simulink model "PMSM3P2LInverterCHILsystem"  (R2026a)
settings: Solver=FixedStepAuto  StopTime=inf  FixedStep=Ts_CPU  EnableMultiTasking=on
undefined symbols (not defined in the file): DiscIntNeverNeededParam, F28379D_ADC_MaxCount, F28379D_ADC_Vmax, Foc_Ki_IxTcpu, Foc_Ki_S, Foc_Kp_I, Foc_Kp_S, Ia_offset, Ib_offset, IO334, IO334_DAC_Vmax, IO334_iDAC_bias, IO334_iDAC_gain, Maxon_645604_J, Maxon_645604_lambda_pm, Maxon_645604_Ld, Maxon_645604_Lq, Maxon_645604_Np, Maxon_645604_Rs, Maxon_645604_StaticF, Maxon_645604_ViscousF, Maxon_Mile_Nslits, PMSM3P2LInverter_limited, PMSM_3P2L_Inverter_Plant, PU_System_I_base, PU_System_N_base, PWM_frequency, Ts_CAN_Tx, Ts_CPU, ts_FPGA_mdl, Ts_UI
libraries: speedgoatlib_hdlCoder_IO3xx x31, mcbcontrolslib x8, canmsglib x6, speedgoatlib_IO611 x3, mcbeeMathTransformLib x3, slpidlib x3, simulink x3, mcbpositiondecoderlib x3, pwm_cpulib x2, mcbhdlplantlib x2, demo_controls x1, quadrature_cpulib x1
(part 1 of 3)
settings Model: DataDictionary=PMSM3P2LInverterDd.sldd  EnableAccessToBaseWorkspace=off  SimulationMode=external  ExtModeEnableFloating=off  Creator=chrisz  LastModifiedBy=mathieu.lu-dac
settings SolverCC: ConcurrentTasks=on  PositivePriorityOrder=on
settings OptimizationCC: ConditionallyExecuteInputs=off  OptimizeBlockIOStorage=off
settings DebuggingCC: AlgebraicLoopMsg=error  SingleTaskRateTransMsg=error  TasksWithSamePriorityMsg=none  ParameterOverflowMsg=warning  ParameterUnderflowMsg=error  FixptConstUnderflowMsg=error  FixptConstOverflowMsg=error
settings HardwareCC: ProdBitPerLong=64.0  ProdHWDeviceType=Intel->x86-64 (Linux 64)  TargetBitPerPointer=64.0  TargetBitPerSizeT=64.0  TargetBitPerPtrDiffT=64.0  TargetLongLongMode=on  TargetIntDivRoundTo=Zero  TargetEndianess=LittleEndian  TargetWordSize=64.0  TargetHWDeviceType=Custom Processor->MATLAB Host Computer
settings RTWCC: SystemTargetFile=speedgoat.tlc  TemplateMakefile=slrealtime_default_tmf  Toolchain=Simulink Real-Time Toolchain  BuildConfiguration=Faster Runs  TargetLang=C++  Description=Speedgoat Real-Time Target Machine
settings SimulinkRealTimeTargetCC: SLRTFileLogMaxRuns=1.0  MultiwordLength=2048.0
settings SimscapeCC: SimscapeNominalValues="[{\"value\":\"1\",\"unit\":\"A\"},{\"value\":\"1\",\"unit\":\"bar\"},{\"value\":\"1\",\"unit\":\"cm^2\"},{\"value\":\"1\",\"unit\":\"cm^3/s\"},{\"value\":\"1\",\"unit\":\"kJ/kg\"},{\"value\":\"1\",\"unit\":\"kW\"},{\"value\":\"1\",\"unit\":\"l\"},{\"value\":\"1\",\"unit\":\"N\"},{\"value\":\"1\",\"unit\":\"N*m\"},{\"value\":\"1\",\"unit\":\"V\"}]"  SimscapeLogType=none  SimscapeLogDataHistory=5000.0

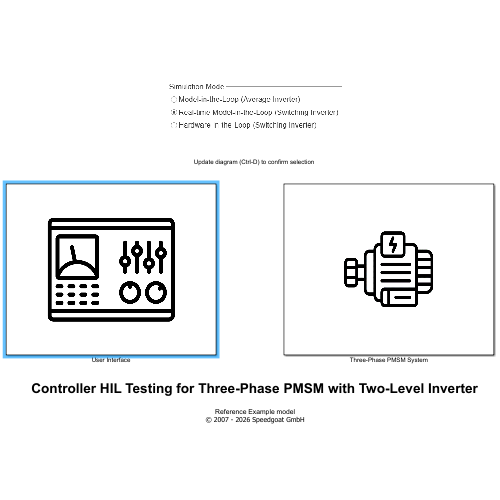
[thumbnail: Simulink's stored preview of the top-level diagram]
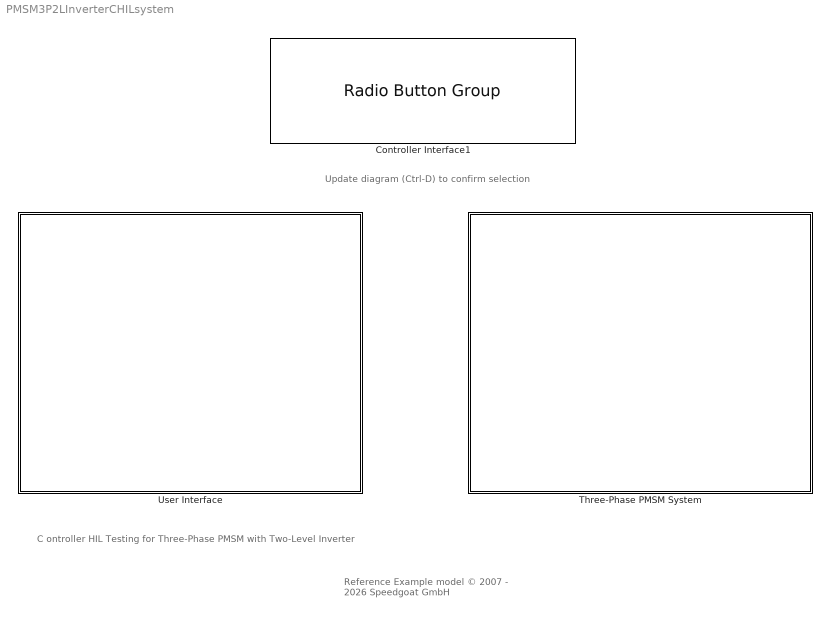
== system PMSM3P2LInverterCHILsystem ==
  note: Update diagram (Ctrl-D) to confirm selection
  note: Reference Example model
      | © 2007 - 2026 Speedgoat GmbH
  note: C ontroller HIL Testing for Three-Phase PMSM with Two-Level Inverter
  Controller Interface1 : RadioButtonGroup  LabelPosition=Hide  SelectedLabel=Real-time Model-in-the-Loop (Switching Inverter)  ButtonGroupName=Simulation Mode
  Three-Phase PMSM System : Subsystem
      mask Display: image('pmsmMask.png'); % Use "Edit Image" on toolstrip to change.
  User Interface : Subsystem
      mask Display: image('UIMask.png');

== system PMSM3P2LInverterCHILsystem/Three-Phase PMSM System ==
  Closed_Loop_FOC : Constant  OutDataTypeStr=boolean  SampleTime=Ts_UI
  Controller : Subsystem  Variant=on  VariantControl=Choice
      settings: PortSchema="{\"entries\":[{\"content\":{\"sides\":[{\"content\":{\"connectorIds\":[\"In1\",\"In2\",\"In3\",\"In4\",\"In5\",\"In6\"]},\"type\":\"ConnectorPlacement.EquallySpacedRectSide\",\"uuid\":\"39f08c92-b87f-4f95-877f-fef0e466fbdb\"},{\"content\":{\"connectorIds\":[\"Out1\"],\"side\":\"RIGHT\"},\"type\":\"ConnectorPlacement.EquallySpacedRectSide\",\"uuid\":\"6fadd6f2-7db3-41c1-89a7-be1692c18c49\"},{\"content\":{\"connectorIds\":[\"Out2\"],\"side\":\"TOP\"},\"type\":\"ConnectorPlacement.EquallySpacedRectSide\",\"uuid\":\"aea4ee68-7094-4bdc-b416-2d8969306971\"}]},\"type\":\"ConnectorPlacement.EquallySpacedConnector\",\"uuid\":\"e129f01f-1291-4735-8ea4-164650c1b4f8\"}],\"packageUris\":[\"http://schema.mathworks.com/mf0/Connector/R2020b\"],\"version\":\"1.0\"}"
      mask Display: image('MCUMask.png');
  Controller Parameters : Subsystem
  Controller_fbk_signals : Subsystem
  EnablePWM : Constant  OutDataTypeStr=boolean  SampleTime=Ts_UI
  Fault Trigering : Subsystem
  Load : Constant  Value=0  OutDataTypeStr=single
  Motor Model Feedback : Subsystem
  Mux : Mux  Inputs=2
  SimulationVariant : Constant  Value=2
  Speed_Cmd_rpm : Constant  Value=500  OutDataTypeStr=single  SampleTime=Ts_UI
  Terminator : Terminator
  Terminator2 : Terminator
  Three-Phase PMSM Drive : Subsystem  Variant=on  VariantControl=Choice
      settings: PortSchema="{\"entries\":[{\"content\":{\"sides\":[{\"content\":{\"connectorIds\":[\"In1\",\"In2\",\"In3\"]},\"type\":\"ConnectorPlacement.EquallySpacedRectSide\",\"uuid\":\"be3bef0c-fa0d-49a9-8d81-4a9438f9f09e\"},{\"content\":{\"connectorIds\":[\"Out1\",\"Out2\",\"Out3\",\"Out4\",\"Out5\",\"Out6\"],\"side\":\"RIGHT\"},\"type\":\"ConnectorPlacement.EquallySpacedRectSide\",\"uuid\":\"a97c4291-bd47-47ae-a87a-e148291abc4a\"},{\"content\":{\"connectorIds\":[\"In4\"],\"side\":\"TOP\"},\"type\":\"ConnectorPlacement.EquallySpacedRectSide\",\"uuid\":\"93bcf0c4-5b44-4ac3-b6c3-6b4577237bd1\"}]},\"type\":\"ConnectorPlacement.EquallySpacedConnector\",\"uuid\":\"9c4ab161-5f4a-4191-8213-47b9045836c1\"}],\"packageUris\":[\"http://schema.mathworks.com/mf0/Connector/R2020b\"],\"version\":\"1.0\"}"
      mask Display: image('pmsmMask.png'); % Use "Edit Image" on toolstrip to change.
  Voltage : Constant  Value=24  OutDataTypeStr=single
  wires:
  Controller/2(Simu_config) -> Three-Phase PMSM Drive/4(Simu_config)
  Voltage/1 -> Three-Phase PMSM Drive/1(V_dc)
  [Iab] -> Controller/1(Iab)
  Closed_Loop_FOC/1 -> Controller/4(Closed_Loop_FOC)
  Controller Parameters/1(Controller Parameters) -> Controller/6(Controller_Parameters)
  Load/1 -> Three-Phase PMSM Drive/3(LdTrq/Spd)
  [QAE_Pos_C] -> Controller/2(QAE_MIL_fbk)
  Mux/1 -> [Iab]
  Fault Trigering/1(Faults) -> Three-Phase PMSM Drive/2(Fault)
  Controller/1(Controller_fbk) -> Controller_fbk_signals/1(Controller_fbk)
  Three-Phase PMSM Drive/1(Ia) -> Mux/1, Motor Model Feedback/1(Ia)
  Three-Phase PMSM Drive/2(Ib) -> Mux/2, Motor Model Feedback/2(Ib)
  Three-Phase PMSM Drive/3(Ic) -> Motor Model Feedback/3(Ic)
  Three-Phase PMSM Drive/4(Motor_Spd) -> Motor Model Feedback/4(Motor_SPD_rads)
  Three-Phase PMSM Drive/6(QAE_Pos_C) -> [QAE_Pos_C]
  Three-Phase PMSM Drive/5(Motor_Angle) -> Terminator/1
  EnablePWM/1 -> Controller/3(EnablePWM)
  Speed_Cmd_rpm/1 -> Controller/5(Speed_CMD_RPM)
  SimulationVariant/1 -> Terminator2/1

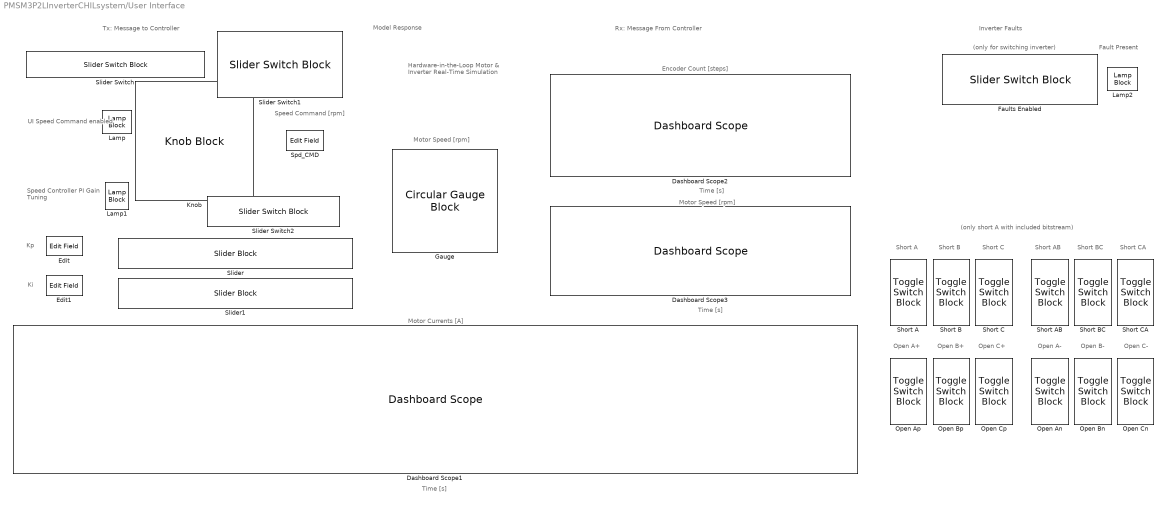
== system PMSM3P2LInverterCHILsystem/User Interface ==
  note: Fault Present
  note: Hardware-in-the-Loop
      | Motor & Inverter
      | Real-Time Simulation
  note: Motor Currents [A]
  note: Model Response
  note: Kp
  note: UI Speed Command
      | enabled
  note: Tx: Message to Controller
  note: Speed Controller
      | PI Gain Tuning
  note: Ki
  note: Rx: Message From Controller
  note: Open A-
  note: Open C-
  note: Short AB
  note: Short B
  note: Short CA
  note: Open A+
  note: Short BC
  note: Open B-
  note: Open B+
  note: Open C+
  note: Short A
  note: Short C
  note: Inverter Faults
  note: Motor Speed [rpm]
  note: Time [s]
  note: Time [s]
  note: Time [s]
  note: Motor Speed [rpm]
  note: Encoder Count [steps]
  note: Speed Command [rpm]
  note: (only for switching inverter)
  note: (only short A with included bitstream)
  Dashboard Scope1 : DashboardScope  ShowInitialText=off  TimeSpan=0.10000000000000001  Ymin=-50  Ymax=50  ScaleAtStop=off  UpdateMode=Scroll  FontColor=[0.0, 0.0, 0.0]
  Dashboard Scope2 : DashboardScope  ShowInitialText=off  TimeSpan=1  Ymin=0  Ymax=1e5  ScaleAtStop=off  FontColor=[0.0, 0.0, 0.0]
  Dashboard Scope3 : DashboardScope  ShowInitialText=off  TimeSpan=10  Ymin=-1500  Ymax=1500  ScaleAtStop=off  FontColor=[0.0, 0.0, 0.0]
  Edit : EditField  LabelPosition=Hide  ShowInitialText=on  Alignment=Center
  Edit1 : EditField  LabelPosition=Hide  ShowInitialText=on  Alignment=Center
  Faults Enabled : SliderSwitchBlock  LabelPosition=Hide
  Gauge : CircularGaugeBlock  LabelPosition=Hide  ScaleMin=-1500  ScaleMax=1500  FontColor=[0.0, 0.0, 0.0]
  Knob : KnobBlock  LabelPosition=Hide  ScaleMin=-1500  ScaleMax=1500
  Lamp : LampBlock  LabelPosition=Hide  DefaultColor=[192.0, 192.0, 192.0]
  Lamp1 : LampBlock  LabelPosition=Hide  DefaultColor=[192.0, 192.0, 192.0]
  Lamp2 : LampBlock  LabelPosition=Hide  DefaultColor=[192.0, 192.0, 192.0]
  Open An : ToggleSwitchBlock  LabelPosition=Hide
  Open Ap : ToggleSwitchBlock  LabelPosition=Hide
  Open Bn : ToggleSwitchBlock  LabelPosition=Hide
  Open Bp : ToggleSwitchBlock  LabelPosition=Hide
  Open Cn : ToggleSwitchBlock  LabelPosition=Hide
  Open Cp : ToggleSwitchBlock  LabelPosition=Hide
  Short A : ToggleSwitchBlock  LabelPosition=Hide
  Short AB : ToggleSwitchBlock  LabelPosition=Hide
  Short B : ToggleSwitchBlock  LabelPosition=Hide
  Short BC : ToggleSwitchBlock  LabelPosition=Hide
  Short C : ToggleSwitchBlock  LabelPosition=Hide
  Short CA : ToggleSwitchBlock  LabelPosition=Hide
  Slider : SliderBlock  LabelPosition=Hide  ScaleMin=1e-5  ScaleMax=10  ScaleType=Log
  Slider Switch : SliderSwitchBlock  LabelPosition=Hide
  Slider Switch1 : SliderSwitchBlock  LabelPosition=Hide
  Slider Switch2 : SliderSwitchBlock  LabelPosition=Hide
  Slider1 : SliderBlock  LabelPosition=Hide  ScaleMin=1e-5  ScaleMax=10  ScaleType=Log
  Spd_CMD : EditField  LabelPosition=Hide  ShowInitialText=on  Alignment=Center

== system PMSM3P2LInverterCHILsystem/Three-Phase PMSM System/Controller ==
  Iab : Inport
  QAE_MIL_fbk : Inport  Port=2
  EnablePWM : Inport  Port=3
  Closed_Loop_FOC : Inport  Port=4
  Speed_CMD_RPM : Inport  Port=5
  Controller_Parameters : Inport  Port=6
  Controller_HIL_CAN : Subsystem  VariantControl=strcmp(get_param([bdroot '/Three-Phase PMSM System/SimulationVariant'], 'Value'),'3')
  Controller_MIL : Subsystem  VariantControl=(default)
  Controller_fbk : Outport
  Simu_config : Outport  Port=2

== system PMSM3P2LInverterCHILsystem/Three-Phase PMSM System/Controller Parameters ==
  Controller_Parameters : BusCreator  Inputs=6
  Controller_Parameters1 : BusCreator  Inputs=6
  Default Values : Constant  OutDataTypeStr=boolean  SampleTime=Ts_UI
  Foc_Ki_S : Constant  Value=Foc_Ki_S  OutDataTypeStr=single
  Foc_Kp_I : Constant  Value=Foc_Kp_I  OutDataTypeStr=single
  Foc_Kp_S : Constant  Value=Foc_Kp_S  OutDataTypeStr=single
  Ia Offset : Constant  Value=Ia_offset  OutDataTypeStr=single
  Ia_offset : Constant  Value=Ia_offset  OutDataTypeStr=single  SampleTime=Ts_UI
  Ib Offset : Constant  Value=Ib_offset  OutDataTypeStr=single
  Ib_offset : Constant  Value=Ib_offset  OutDataTypeStr=single  SampleTime=Ts_UI
  Ki_S : Constant  Value=0.1  OutDataTypeStr=single  SampleTime=Ts_UI
  Ki_i*Tcpu : Constant  Value=Foc_Ki_IxTcpu  OutDataTypeStr=single  SampleTime=Ts_UI
  Ki_i*Tcpu1 : Constant  Value=Foc_Ki_IxTcpu  OutDataTypeStr=single
  Kp_I : Constant  Value=Foc_Kp_I  OutDataTypeStr=single  SampleTime=Ts_UI
  Kp_S : Constant  Value=0.1  OutDataTypeStr=single  SampleTime=Ts_UI
  Rate Transition : RateTransition  OutPortSampleTime=Ts_UI
  Switch : Switch  Criteria=u2 ~= 0  SaturateOnIntegerOverflow=off  InputSameDT=off
  Controller Parameters : Outport
  wires:
  Ia_offset/1 -> Controller_Parameters/5  "Ia_offset"
  Foc_Kp_S/1 -> Controller_Parameters1/1  "Kp_S"
  Ia Offset/1 -> Controller_Parameters1/5  "Ia_offset"
  Ib Offset/1 -> Controller_Parameters1/6  "Ib_offset"
  Controller_Parameters/1 -> Switch/3
  Foc_Ki_S/1 -> Controller_Parameters1/2  "Ki_S"
  Foc_Kp_I/1 -> Controller_Parameters1/3  "Kp_I"
  Controller_Parameters1/1 -> Rate Transition/1
  Ib_offset/1 -> Controller_Parameters/6  "Ib_offset"
  Ki_i*Tcpu/1 -> Controller_Parameters/4  "Ki_IxTcpu"
  Ki_S/1 -> Controller_Parameters/2  "Ki_S"
  Ki_i*Tcpu1/1 -> Controller_Parameters1/4  "Ki_IxTcpu"
  Kp_I/1 -> Controller_Parameters/3  "Kp_I"
  Kp_S/1 -> Controller_Parameters/1  "Kp_S"
  Switch/1 -> Controller Parameters/1
  Rate Transition/1 -> Switch/1
  Default Values/1 -> Switch/2  "Default Values"

== system PMSM3P2LInverterCHILsystem/Three-Phase PMSM System/Controller_fbk_signals ==
  Controller_fbk : Inport
  Data Type Conversion : DataTypeConversion  OutDataTypeStr=boolean  SaturateOnIntegerOverflow=off  RndMeth=Floor
  Demux : Demux
  Terminator{,1..3} (4 alike) : Terminator
  wires:
  Demux/1 -> Terminator1/1  "Speed_fbk"
  Controller_fbk/1 -> Demux/1
  Demux/2 -> Terminator3/1  "Encoder_Pos_fbk"
  Demux/4 -> Data Type Conversion/1  "Spd_Pot_fdk"
  Demux/3 -> Terminator2/1  "Speed_Cmd_fbk"
  Data Type Conversion/1 -> Terminator/1  "Spd_pot_enable"

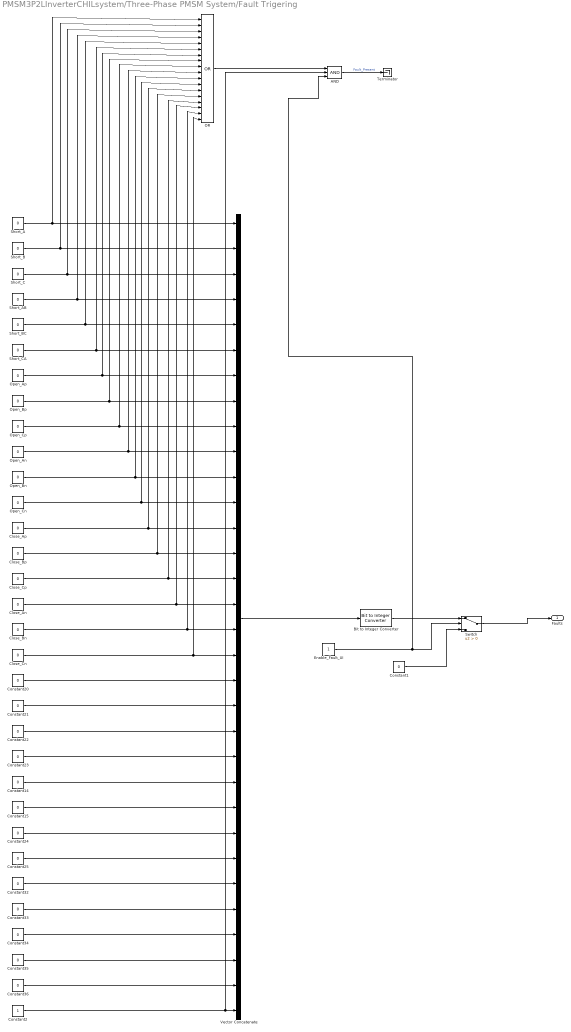
== system PMSM3P2LInverterCHILsystem/Three-Phase PMSM System/Fault Trigering ==
  AND : Logic  Inputs=3  IconShape=distinctive  AllPortsSameDT=off  OutDataTypeStr=boolean
  Bit to Integer Converter : simulink/Logic and Bit Operations/Bit to Integer Converter  nbits=32  bitOrder=LSB first  signedOutputValues=Unsigned  outDtype=uint32  outDtypeSigned=Inherit via internal rule
  Close_An : Constant  Value=0  OutDataTypeStr=boolean  SampleTime=Ts_UI
  Close_Ap : Constant  Value=0  OutDataTypeStr=boolean  SampleTime=Ts_UI
  Close_Bn : Constant  Value=0  OutDataTypeStr=boolean  SampleTime=Ts_UI
  Close_Bp : Constant  Value=0  OutDataTypeStr=boolean  SampleTime=Ts_UI
  Close_Cn : Constant  Value=0  OutDataTypeStr=boolean  SampleTime=Ts_UI
  Close_Cp : Constant  Value=0  OutDataTypeStr=boolean  SampleTime=Ts_UI
  Constant1 : Constant  Value=0  OutDataTypeStr=uint32
  Constant{14..15,20..25,32..36} (13 alike) : Constant  Value=0  OutDataTypeStr=boolean  SampleTime=Ts_UI
  Constant2 : Constant  OutDataTypeStr=boolean  SampleTime=Ts_UI
  Enable_Fault_UI : Constant  OutDataTypeStr=boolean  SampleTime=Ts_UI
  OR : Logic  Operator=OR  Inputs=18  IconShape=distinctive  AllPortsSameDT=off  OutDataTypeStr=boolean
  Open_An : Constant  Value=0  OutDataTypeStr=boolean  SampleTime=Ts_UI
  Open_Ap : Constant  Value=0  OutDataTypeStr=boolean  SampleTime=Ts_UI
  Open_Bn : Constant  Value=0  OutDataTypeStr=boolean  SampleTime=Ts_UI
  Open_Bp : Constant  Value=0  OutDataTypeStr=boolean  SampleTime=Ts_UI
  Open_Cn : Constant  Value=0  OutDataTypeStr=boolean  SampleTime=Ts_UI
  Open_Cp : Constant  Value=0  OutDataTypeStr=boolean  SampleTime=Ts_UI
  Short_A : Constant  Value=0  OutDataTypeStr=boolean  SampleTime=Ts_UI
  Short_AB : Constant  Value=0  OutDataTypeStr=boolean  SampleTime=Ts_UI
  Short_B : Constant  Value=0  OutDataTypeStr=boolean  SampleTime=Ts_UI
  Short_BC : Constant  Value=0  OutDataTypeStr=boolean  SampleTime=Ts_UI
  Short_C : Constant  Value=0  OutDataTypeStr=boolean  SampleTime=Ts_UI
  Short_CA : Constant  Value=0  OutDataTypeStr=boolean  SampleTime=Ts_UI
  Switch : Switch  Criteria=u2 > Threshold  SaturateOnIntegerOverflow=off  InputSameDT=off
  Terminator : Terminator
  Vector Concatenate : Concatenate  NumInputs=32
  Faults : Outport
  wires:
  Open_Cn/1 -> OR/12, Vector Concatenate/12
  Open_Cp/1 -> OR/9, Vector Concatenate/9
  Short_A/1 -> OR/1, Vector Concatenate/1
  Open_Bp/1 -> OR/8, Vector Concatenate/8
  Short_B/1 -> Vector Concatenate/2, OR/2
  Short_C/1 -> Vector Concatenate/3, OR/3
  Short_AB/1 -> Vector Concatenate/4, OR/4
  Short_BC/1 -> Vector Concatenate/5, OR/5
  Short_CA/1 -> OR/6, Vector Concatenate/6
  Constant36/1 -> Vector Concatenate/31
  Open_Bn/1 -> OR/11, Vector Concatenate/11
  Open_An/1 -> OR/10, Vector Concatenate/10
  Open_Ap/1 -> OR/7, Vector Concatenate/7
  Close_An/1 -> OR/16, Vector Concatenate/16
  Close_Ap/1 -> OR/13, Vector Concatenate/13
  Close_Cn/1 -> OR/18, Vector Concatenate/18
  Close_Bn/1 -> OR/17, Vector Concatenate/17
  Close_Cp/1 -> OR/15, Vector Concatenate/15
  Close_Bp/1 -> OR/14, Vector Concatenate/14
  Constant15/1 -> Vector Concatenate/24
  Constant14/1 -> Vector Concatenate/23
  Constant21/1 -> Vector Concatenate/20
  Constant20/1 -> Vector Concatenate/19
  Constant25/1 -> Vector Concatenate/26
  Constant24/1 -> Vector Concatenate/25
  Constant23/1 -> Vector Concatenate/22
  Constant22/1 -> Vector Concatenate/21
  Constant35/1 -> Vector Concatenate/30
  Constant34/1 -> Vector Concatenate/29
  Constant33/1 -> Vector Concatenate/28
  Constant32/1 -> Vector Concatenate/27
  Enable_Fault_UI/1 -> AND/3, Switch/2
  Vector Concatenate/1 -> Bit to Integer Converter/1
  Switch/1 -> Faults/1
  Bit to Integer Converter/1 -> Switch/1
  Constant1/1 -> Switch/3
  OR/1 -> AND/1
  AND/1 -> Terminator/1  "Fault_Present"
  Constant2/1 -> AND/2, Vector Concatenate/32

== system PMSM3P2LInverterCHILsystem/Three-Phase PMSM System/Motor Model Feedback ==
  Ia : Inport
  Ib : Inport  Port=2
  Ic : Inport  Port=3
  Motor_SPD_rads : Inport  Port=4
  Rate Transition{,1..3} (4 alike) : RateTransition  OutPortSampleTime=Ts_UI_fast
  Terminator{,1..3} (4 alike) : Terminator
  radsTOrpm : Gain  Gain=60/(2*pi)
  wires:
  Rate Transition1/1 -> Terminator/1  "Ia"
  Rate Transition3/1 -> Terminator2/1  "Ic"
  Rate Transition2/1 -> Terminator1/1  "Ib"
  Ib/1 -> Rate Transition2/1
  Ia/1 -> Rate Transition1/1
  Ic/1 -> Rate Transition3/1
  Motor_SPD_rads/1 -> Rate Transition/1
  radsTOrpm/1 -> Terminator3/1  "Motor Speed RPM"
  Rate Transition/1 -> radsTOrpm/1

== system PMSM3P2LInverterCHILsystem/Three-Phase PMSM System/Three-Phase PMSM Drive ==
  V_dc : Inport
  Fault : Inport  Port=2
  LdTrq/Spd : Inport  Port=3
  Simu_config : Inport  Port=4
  PMSM and average inverter : Subsystem  VariantControl=str2num(get_param([bdroot '/Three-Phase PMSM System/SimulationVariant'], 'Value'))==1
  PMSM and inverter with switching dynamics : Subsystem  VariantControl=str2num(get_param([bdroot '/Three-Phase PMSM System/SimulationVariant'], 'Value'))>1
  Ia : Outport
  Ib : Outport  Port=2
  Ic : Outport  Port=3
  Motor_Spd : Outport  Port=4
  Motor_Angle : Outport  Port=5
  QAE_Pos_C : Outport  Port=6

== system PMSM3P2LInverterCHILsystem/Three-Phase PMSM System/Controller/Controller_HIL_CAN ==
  Iab : Inport
  QAE_MIL_fbk : Inport  Port=2
  EnablePWM : Inport  Port=3
  Closed_Loop_FOC : Inport  Port=4
  Speed_CMD_RPM : Inport  Port=5
  Controller_Parameters : Inport  Port=6
  CAN Communication 611 : Subsystem
  Data Type Conversion : DataTypeConversion  OutDataTypeStr=uint8  SaturateOnIntegerOverflow=off  RndMeth=Floor
  Data Type Conversion1 : DataTypeConversion  OutDataTypeStr=uint8  SaturateOnIntegerOverflow=off  RndMeth=Floor
  Data Type Conversion2 : DataTypeConversion  OutDataTypeStr=single  SaturateOnIntegerOverflow=off  RndMeth=Floor
  Internal PWM configuration1 : Subsystem
  Mux : Mux
  Terminator8 : Terminator
  Terminator9 : Terminator
  Simu_config : Outport
  Controller_fbk : Outport  Port=2
  wires:
  Iab/1 -> Terminator9/1
  Speed_CMD_RPM/1 -> CAN Communication 611/1(Speed_CMD_rpm)
  Controller_Parameters/1 -> CAN Communication 611/4(Controller_Parameters)
  EnablePWM/1 -> Data Type Conversion1/1
  Data Type Conversion/1 -> CAN Communication 611/2(Closed_loop)
  QAE_MIL_fbk/1 -> Terminator8/1
  Closed_Loop_FOC/1 -> Data Type Conversion/1
  Data Type Conversion1/1 -> CAN Communication 611/3(EnablePWM)
  Data Type Conversion2/1 -> Controller_fbk/1
  CAN Communication 611/2(Pos_fdk) -> Mux/2
  CAN Communication 611/1(Speed_fbk) -> Mux/1
  CAN Communication 611/4(Spd_pot) -> Mux/4
  CAN Communication 611/3(Speed_Cmd) -> Mux/3
  Mux/1 -> Data Type Conversion2/1
  Internal PWM configuration1/1(Simu Config) -> Simu_config/1

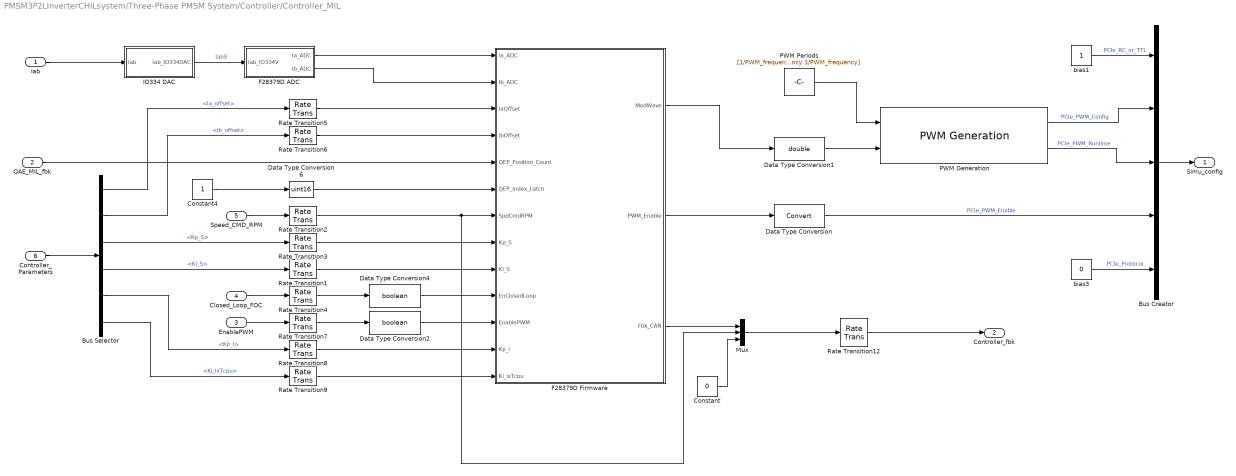
== system PMSM3P2LInverterCHILsystem/Three-Phase PMSM System/Controller/Controller_MIL ==
  Iab : Inport
  QAE_MIL_fbk : Inport  Port=2
  EnablePWM : Inport  Port=3
  Closed_Loop_FOC : Inport  Port=4
  Speed_CMD_RPM : Inport  Port=5
  Controller_Parameters : Inport  Port=6
  Bus Creator : BusCreator  Inputs=5
  Bus Selector : BusSelector  OutputSignals=Ia_offset,Ib_offset,Kp_S,Ki_S,Kp_I,Ki_IxTcpu
  Constant : Constant  Value=0  OutDataTypeStr=single  SampleTime=Ts_CPU
  Constant4 : Constant
  Data Type Conversion : DataTypeConversion  SaturateOnIntegerOverflow=off  RndMeth=Floor
  Data Type Conversion1 : DataTypeConversion  OutDataTypeStr=double  SaturateOnIntegerOverflow=off  RndMeth=Floor
  Data Type Conversion2 : DataTypeConversion  OutDataTypeStr=boolean  SaturateOnIntegerOverflow=off  RndMeth=Floor
  Data Type Conversion4 : DataTypeConversion  OutDataTypeStr=boolean  SaturateOnIntegerOverflow=off  RndMeth=Floor
  Data Type Conversion6 : DataTypeConversion  OutDataTypeStr=uint16  RndMeth=Simplest  SaturateOnIntegerOverflow=off
  F28379D ADC : Subsystem
  F28379D Firmware : Subsystem
  IO334 DAC : Subsystem
  Mux : Mux  Inputs=3
  PWM Generation : pwm_cpulib/PWM Generation  f_FPGA=f_FPGA  n_channels=3  sel_scaling=CPU  protection_param=A/B are forced off when A/B are on.  deadband_sec=0  natural_update=At period starts  delay=0  trigger_duration_sec=[1e-6]  trigger_period_start=off  trigger_half_of_the_period=off  trigger_a_on=off  trigger_a_off=off  trigger_b_on=off  trigger_b_off=off  bit_width_pwm_gen=24  invert_a=off  invert_b=off  invert_c=off  showPhaseInput=off
      settings: SourceProductName=PWM CPU Library
  PWM Periods : Constant  Value=[1/PWM_frequency 1/PWM_frequency 1/PWM_frequency]  OutDataTypeStr=double  SampleTime=-1
  Rate Transition1 : RateTransition  OutPortSampleTime=Ts_speed
  Rate Transition12 : RateTransition  OutPortSampleTime=Ts_UI
  Rate Transition{2,5..9} (6 alike) : RateTransition  OutPortSampleTime=Ts_CPU
  Rate Transition3 : RateTransition  OutPortSampleTime=Ts_speed
  Rate Transition4 : RateTransition  InitialCondition=1  OutPortSampleTime=Ts_CPU
  bias1 : Constant  OutDataTypeStr=boolean  SampleTime=Ts_CPU
  bias3 : Constant  Value=0  OutDataTypeStr=boolean  SampleTime=Ts_CPU
  Simu_config : Outport
  Controller_fbk : Outport  Port=2
  wires:
  bias1/1 -> Bus Creator/1  "PCIe_RC_or_TTL"
  Bus Creator/1 -> Simu_config/1
  Constant4/1 -> Data Type Conversion6/1
  Data Type Conversion/1 -> Bus Creator/4  "PCIe_PWM_Enable"
  Iab/1 -> IO334 DAC/1(Iab)
  IO334 DAC/1(Iab_IO334DAC) -> F28379D ADC/1(Iab_IO334V)  "IabV"
  F28379D ADC/1(Ia_ADC) -> F28379D Firmware/1(Ia_ADC)
  F28379D ADC/2(Ib_ADC) -> F28379D Firmware/2(Ib_ADC)
  QAE_MIL_fbk/1 -> F28379D Firmware/5(QEP_Position_Count)
  Data Type Conversion6/1 -> F28379D Firmware/6(QEP_Index_Latch)
  Bus Selector/3 -> Rate Transition3/1  "<Kp_S>"
  F28379D Firmware/2(PWM_Enable) -> Data Type Conversion/1
  Data Type Conversion2/1 -> F28379D Firmware/11(EnablePWM)
  Data Type Conversion4/1 -> F28379D Firmware/10(EnClosedLoop)
  Bus Selector/4 -> Rate Transition1/1  "<Ki_S>"
  Closed_Loop_FOC/1 -> Rate Transition4/1
  Controller_Parameters/1 -> Bus Selector/1
  Bus Selector/1 -> Rate Transition5/1  "<Ia_offset>"
  Bus Selector/2 -> Rate Transition6/1  "<Ib_offset>"
  Bus Selector/5 -> Rate Transition8/1  "<Kp_I>"
  Bus Selector/6 -> Rate Transition9/1  "<Ki_IxTcpu>"
  EnablePWM/1 -> Rate Transition7/1
  Mux/1 -> Rate Transition12/1
  F28379D Firmware/3(Fbk_CAN) -> Mux/1
  Speed_CMD_RPM/1 -> Rate Transition2/1
  Rate Transition3/1 -> F28379D Firmware/8(Kp_S)
  Rate Transition1/1 -> F28379D Firmware/9(Ki_S)
  Rate Transition5/1 -> F28379D Firmware/3(IaOffset)
  Rate Transition6/1 -> F28379D Firmware/4(IbOffset)
  Rate Transition4/1 -> Data Type Conversion4/1
  Rate Transition7/1 -> Data Type Conversion2/1
  Rate Transition8/1 -> F28379D Firmware/12(Kp_i)
  Rate Transition9/1 -> F28379D Firmware/13(Ki_ixTcpu)
  Rate Transition12/1 -> Controller_fbk/1
  Constant/1 -> Mux/3
  Rate Transition2/1 -> F28379D Firmware/7(SpdCmdRPM), Mux/2
  bias3/1 -> Bus Creator/5  "PCIe_Protocol"
  PWM Periods/1 -> PWM Generation/1
  PWM Generation/1 -> Bus Creator/2  "PCIe_PWM_Config"
  PWM Generation/2 -> Bus Creator/3  "PCIe_PWM_Runtime"
  Data Type Conversion1/1 -> PWM Generation/2
  F28379D Firmware/1(ModWave) -> Data Type Conversion1/1

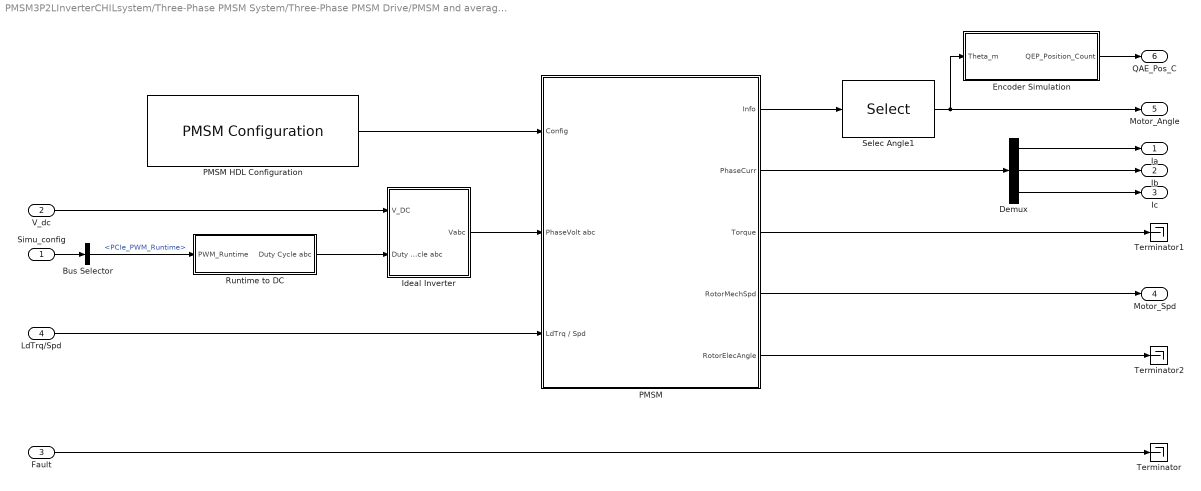
== system PMSM3P2LInverterCHILsystem/Three-Phase PMSM System/Three-Phase PMSM Drive/PMSM and average inverter ==
  Simu_config : Inport
  V_dc : Inport  Port=2
  Fault : Inport  Port=3
  LdTrq/Spd : Inport  Port=4
  Bus Selector : BusSelector  OutputSignals=PCIe_PWM_Runtime
  Demux : Demux  Outputs=3
  Encoder Simulation : Subsystem
  Ideal Inverter : Subsystem
  PMSM : Subsystem
  PMSM HDL Configuration : mcbhdlplantlib/PMSM Configuration  portConfig=Torque  Trq_N_mode=0  outDataTypePop=Floating-point  outWordLength=32  Pp=Maxon_645604_Np  Rs=Maxon_645604_Rs  Ld=Maxon_645604_Ld  Lq=Maxon_645604_Lq  lambda_pm=Maxon_645604_lambda_pm  J=Maxon_645604_J  B=Maxon_645604_ViscousF*100  f=Maxon_645604_StaticF
  Runtime to DC : Subsystem
  Selec Angle1 : Selector  InputPortWidth=14  IndexOptions=Index vector (dialog)  Indices=[10]  OutputSizes=1
  Terminator : Terminator
  Terminator1 : Terminator
  Terminator2 : Terminator
  Ia : Outport
  Ib : Outport  Port=2
  Ic : Outport  Port=3
  Motor_Spd : Outport  Port=4
  Motor_Angle : Outport  Port=5
  QAE_Pos_C : Outport  Port=6
  wires:
  PMSM/4(RotorMechSpd) -> Motor_Spd/1
  Demux/2 -> Ib/1
  Selec Angle1/1 -> Motor_Angle/1, Encoder Simulation/1(Theta_m)
  Demux/3 -> Ic/1
  LdTrq/Spd/1 -> PMSM/3(LdTrq / Spd)
  PMSM/2(PhaseCurr) -> Demux/1
  Demux/1 -> Ia/1
  Ideal Inverter/1(Vabc) -> PMSM/2(PhaseVolt abc)
  V_dc/1 -> Ideal Inverter/1(V_DC)
  Simu_config/1 -> Bus Selector/1
  Fault/1 -> Terminator/1
  Encoder Simulation/1(QEP_Position_Count) -> QAE_Pos_C/1
  PMSM/3(Torque) -> Terminator1/1
  PMSM/5(RotorElecAngle) -> Terminator2/1
  PMSM/1(Info) -> Selec Angle1/1
  Bus Selector/1 -> Runtime to DC/1(PWM_Runtime)  "<PCIe_PWM_Runtime>"
  Runtime to DC/1(Duty Cycle abc) -> Ideal Inverter/2(Duty Cycle abc)
  PMSM HDL Configuration/1 -> PMSM/1(Config)

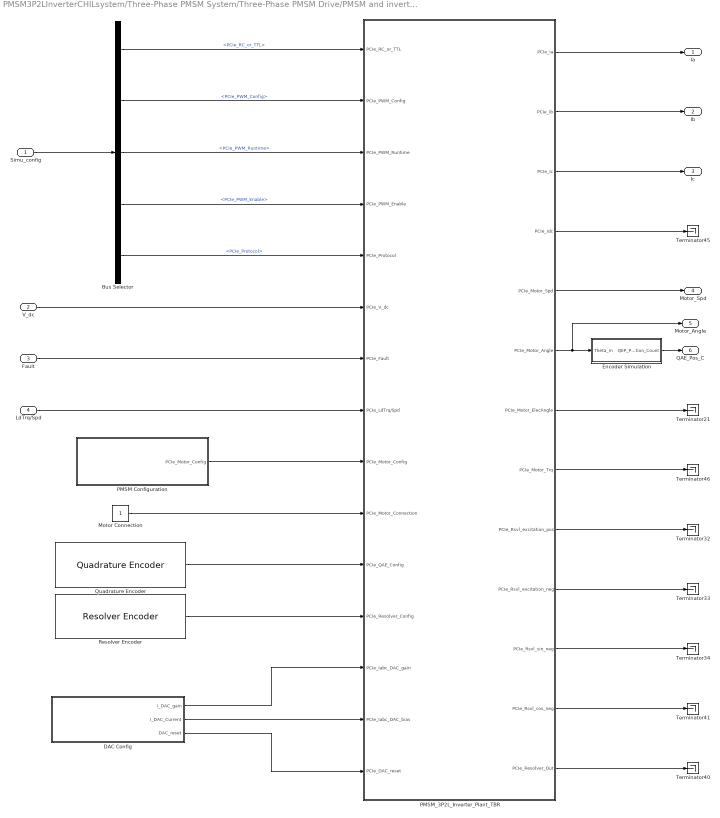
== system PMSM3P2LInverterCHILsystem/Three-Phase PMSM System/Three-Phase PMSM Drive/PMSM and inverter with switching dynamics ==
  Simu_config : Inport
  V_dc : Inport  Port=2
  Fault : Inport  Port=3
  LdTrq/Spd : Inport  Port=4
  Bus Selector : BusSelector  OutputSignals=PCIe_RC_or_TTL,PCIe_PWM_Config,PCIe_PWM_Runtime,PCIe_PWM_Enable,PCIe_Protocol
  DAC Config : Subsystem
  Encoder Simulation : Subsystem
  Motor Connection : Constant  OutDataTypeStr=boolean
  PMSM Configuration : Subsystem  InitFcn=|  mask(PMSM Configuration){portConfig=Torque, Trq_N_mode=0, Ts=Ts_CPU, Pp=Maxon_645604_Np, Rs=Maxon_645604_Rs, Ld=Maxon_645604_Ld, Lq=Maxon_645604_Lq, lambda_pm=Maxon_645604_lambda_pm, J=Maxon_645604_J, B=Maxon_645604_ViscousF*100, f=Maxon_645604_StaticF}
      | mcb.internal.manageMCBResource('register',gcbh);
      | mcb.internal.logDDUXData;
      mask prompts: portConfig "mcb:PlantLib:CfgMechInCfg"; Ts "mcb:PlantLib:CfgTs"; Pp "mcb:PlantLib:PMSMCfgPp"; Rs "mcb:PlantLib:PMSMCfgRs"; Ld "mcb:PlantLib:PMSMCfgLd"; Lq "mcb:PlantLib:PMSMCfgLq"; lambda_pm "mcb:PlantLib:PMSMCfgLambda"; J "mcb:PlantLib:PMSMCfgJ"; B "mcb:PlantLib:PMSMCfgB"; f "mcb:PlantLib:PMSMCfgf"
      mask help: mcb:PlantLib:PMSMCfgDes
      mask Help: eval('mcb_helpview(''pmsmhdlconfig'')')
      mask TypeOptions portConfig: mcb:PlantLib:CfgTorque | mcb:PlantLib:CfgSpd
      mask Callback portConfig:
      | %Do not run initialization code if model is running
      | invalidStatus = {'external','running','compiled','restarting','paused','terminating'};
      | if ~any(strcmpi(get_param(bdroot(gcb),'SimulationStatus'),invalidStatus))
      |     % Check the value selected in the pop-up
      |     mask = Simulink.Mask.get(gcb);
      |     portConfigStr = get_param(gcb, 'portConfig');
      |     if strcmp(portConfigStr, 'Torque')
      |         % Set Trq_N_mode value to 0
      |         mask.getParameter('Trq_N_mode').Value = '0';
      | 
      |     elseif strcmp(portConfigStr, 'Speed')
      |         % Set Trq_N_mode value to 2
      |         mask.getParameter('Trq_N_mode').Value = '1';
      | 
      |     end
      | end
      mask DialogControl DescGroupVar Prompt: mcb:PlantLib:PMSMCfgTitle
      mask DialogControl ParameterGroupVar Prompt: mcb:PlantLib:CfgBlk
      mask DialogControl portConfig Prompt: Mechanical input configuration:
      mask DialogControl Ts Prompt: Sample time (s):
      mask DialogControl Container4 Prompt: mcb:PlantLib:CfgParam
      mask DialogControl Pp Prompt: Number of pole pairs:
      mask DialogControl Rs Prompt: Stator resistance per phase (Ohm):
      mask DialogControl Ld Prompt: Stator d-axis inductance (H):
      mask DialogControl Lq Prompt: Stator q-axis inductance (H):
      mask DialogControl lambda_pm Prompt: Permanent flux linkage constant (Wb):
      mask DialogControl J Prompt: Inertia (kgm^2):
      mask DialogControl B Prompt: Viscous damping (Nm/rad/s):
      mask DialogControl f Prompt: Static friction (Nm):
      mask Display:
      | disp('PMSM\nConfiguration');
      | port_label('output',1,'Config');
  PMSM_3P2L_Inverter_Plant_TBR : Subsystem
      mask Display: disp('Plant Bitstream Block')
  Quadrature Encoder : quadrature_cpulib/Quadrature Encoder  FPGA_freq=f_FPGA  n_channels=[1]  sel_scaling=FPGA  useSpeed=off  usePosition=on  numOfSlots=Maxon_Mile_Nslits  sigAswitchOn=[180]  sigBswitchOff=[90]  sigBswitchOn=[270]  sigAdismissEn=off  sigAdismissSingle=on  sigAdismissHigh=on  sigBdismissEn=off  sigBdismissSingle=on  sigBdismissHigh=on
      settings: SourceProductName=Quadrature CPU Library
  Resolver Encoder : resolver_cpulib/Resolver Encoder  Ts=Ts_UI  ts_resolver=ts_FPGA_mdl  n_channels=1  sel_scaling=FPGA  useSpeed=on  usePosition=off  pole_pairs=1  gain_dynamic=off  gainVector=[1, 1, 1, 1]  offset_dynamic=off  offsetVector=[0, 0, 0, 0]  exct_freq=2  angle_offset=0  exct_amplitude=10  position_init_enb=off  rotor_position=90  int_exct_enb=off  exct_out_enb=off  phase_delay=0  time_step_delay=0  adcRange=2.5  dacRange=2.5
      settings: SourceProductName=Resolver CPU Library
  Terminator{21,32..34,40..41,45..46} (8 alike) : Terminator
  Ia : Outport
  Ib : Outport  Port=2
  Ic : Outport  Port=3
  Motor_Spd : Outport  Port=4
  Motor_Angle : Outport  Port=5
  QAE_Pos_C : Outport  Port=6
  wires:
  PMSM_3P2L_Inverter_Plant_TBR/10(PCIe_Rsvl_excitation_neg) -> Terminator33/1
  DAC Config/1(I_DAC_gain) -> PMSM_3P2L_Inverter_Plant_TBR/13(PCIe_Iabc_DAC_gain)
  DAC Config/3(DAC_reset) -> PMSM_3P2L_Inverter_Plant_TBR/15(PCIe_DAC_reset)
  PMSM_3P2L_Inverter_Plant_TBR/7(PCIe_Motor_ElecAngle) -> Terminator21/1
  PMSM_3P2L_Inverter_Plant_TBR/12(PCIe_Rsvl_cos_neg) -> Terminator41/1
  PMSM_3P2L_Inverter_Plant_TBR/13(PCIe_Resolver_Out) -> Terminator40/1
  V_dc/1 -> PMSM_3P2L_Inverter_Plant_TBR/6(PCIe_V_dc)
  PMSM_3P2L_Inverter_Plant_TBR/8(PCIe_Motor_Trq) -> Terminator46/1
  Resolver Encoder/1 -> PMSM_3P2L_Inverter_Plant_TBR/12(PCIe_Resolver_Config)
  PMSM_3P2L_Inverter_Plant_TBR/4(PCIe_Idc) -> Terminator45/1
  Quadrature Encoder/1 -> PMSM_3P2L_Inverter_Plant_TBR/11(PCIe_QAE_Config)
  Motor Connection/1 -> PMSM_3P2L_Inverter_Plant_TBR/10(PCIe_Motor_Connection)
  PMSM_3P2L_Inverter_Plant_TBR/9(PCIe_Rsvl_excitation_pos) -> Terminator32/1
  Fault/1 -> PMSM_3P2L_Inverter_Plant_TBR/7(PCIe_Fault)
  PMSM_3P2L_Inverter_Plant_TBR/11(PCIe_Rsvl_sin_neg) -> Terminator34/1
  DAC Config/2(I_DAC_Current) -> PMSM_3P2L_Inverter_Plant_TBR/14(PCIe_Iabc_DAC_bias)
  Simu_config/1 -> Bus Selector/1
  Bus Selector/4 -> PMSM_3P2L_Inverter_Plant_TBR/4(PCIe_PWM_Enable)  "<PCIe_PWM_Enable>"
  Bus Selector/5 -> PMSM_3P2L_Inverter_Plant_TBR/5(PCIe_Protocol)  "<PCIe_Protocol>"
  Bus Selector/1 -> PMSM_3P2L_Inverter_Plant_TBR/1(PCIe_RC_or_TTL)  "<PCIe_RC_or_TTL>"
  LdTrq/Spd/1 -> PMSM_3P2L_Inverter_Plant_TBR/8(PCIe_LdTrq/Spd)
  PMSM_3P2L_Inverter_Plant_TBR/3(PCIe_Ic) -> Ic/1
  PMSM_3P2L_Inverter_Plant_TBR/6(PCIe_Motor_Angle) -> Motor_Angle/1, Encoder Simulation/1(Theta_m)
  PMSM_3P2L_Inverter_Plant_TBR/5(PCIe_Motor_Spd) -> Motor_Spd/1
  PMSM_3P2L_Inverter_Plant_TBR/2(PCIe_Ib) -> Ib/1
  Encoder Simulation/1(QEP_Position_Count) -> QAE_Pos_C/1
  PMSM_3P2L_Inverter_Plant_TBR/1(PCIe_Ia) -> Ia/1
  Bus Selector/3 -> PMSM_3P2L_Inverter_Plant_TBR/3(PCIe_PWM_Runtime)  "<PCIe_PWM_Runtime>"
  Bus Selector/2 -> PMSM_3P2L_Inverter_Plant_TBR/2(PCIe_PWM_Config)  "<PCIe_PWM_Config>"
  PMSM Configuration/1(PCIe_Motor_Config) -> PMSM_3P2L_Inverter_Plant_TBR/9(PCIe_Motor_Config)

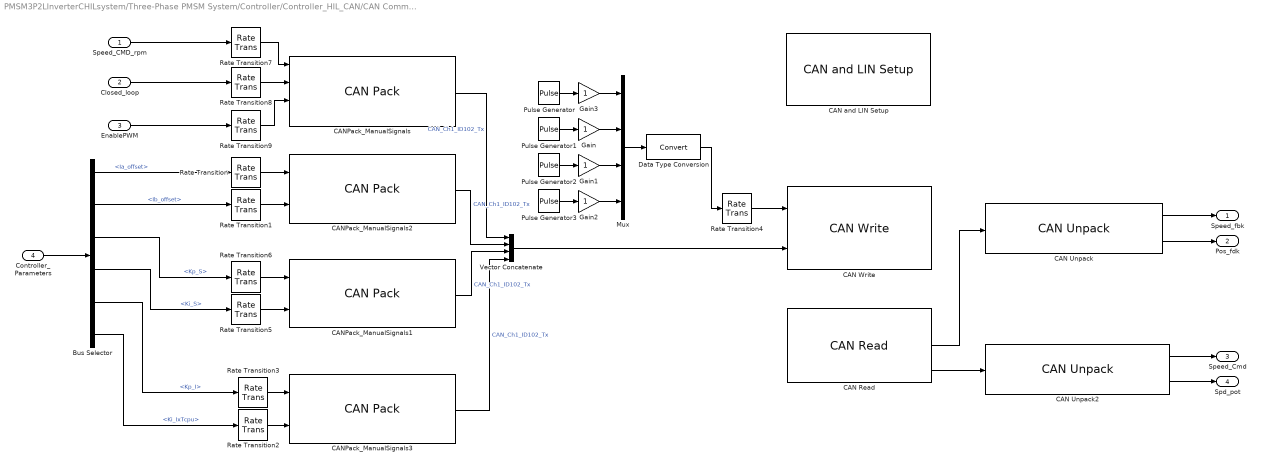
== system PMSM3P2LInverterCHILsystem/Three-Phase PMSM System/Controller/Controller_HIL_CAN/CAN Communication 611 ==
  Speed_CMD_rpm : Inport
  Closed_loop : Inport  Port=2
  EnablePWM : Inport  Port=3
  Controller_Parameters : Inport  Port=4
  Bus Selector : BusSelector  OutputSignals=Ia_offset,Ib_offset,Kp_S,Ki_S,Kp_I,Ki_IxTcpu
  "CAN Read " : speedgoatlib_IO611/CAN Read   moduleType=IO611  id=1  channel=1  canType=CAN (HS)  useBusOut=on  HasMulRead=Specify by IDs  MsgIDlist=[1 2]  isEFF=off  LabelInHex=on  enableInput=off  ts=1e-3  initValues=[611 1 0.001 0 1 1 0 1 0 2 2 1 2]
      settings: SourceProductName=IO611
  CAN Unpack : canmsglib/CAN Unpack  MsgList=(none)  MsgName=Speed_TI_Out  MsgIDType=Standard (11-bit identifier)  MsgIdentifier=1  MsgLength=8  SignalInfo={ 'Speed_fbk', '0', '32', 'LE', 'single', 'Standard', '0', '1', '0', '-Inf', 'Inf'; 'Pos_fbk', '32', '32', 'LE', 'single', 'Standard', '0', '1', '0', '-Inf', 'Inf' }  IDPort=off  TimestampPort=off  ErrorPort=off  RemotePort=off  LengthPort=off  StatusPort=off  ApplyMinMax=off
  CAN Unpack2 : canmsglib/CAN Unpack  MsgList=(none)  MsgName=Speed_Cmd_fbk  MsgIDType=Standard (11-bit identifier)  MsgIdentifier=2  MsgLength=8  SignalInfo={ 'Speed_Cmd', '0', '32', 'LE', 'single', 'Standard', '0', '1', '0', '-Inf', 'Inf'; 'Spd_pot', '32', '32', 'LE', 'single', 'Standard', '0', '1', '0', '-Inf', 'Inf' }  IDPort=off  TimestampPort=off  ErrorPort=off  RemotePort=off  LengthPort=off  StatusPort=off  ApplyMinMax=off
  "CAN Write " : speedgoatlib_IO611/CAN Write   moduleType=IO611  id=1  channel=1  canType=CAN (HS)  useBusIn=on  numOfMsg=4  enableInput=on  enableStatusPort=off  initValues=[611 1 0.2 0 1 1 0 4 1 1]  ts=Ts_CAN_Tx
      settings: SourceProductName=IO611
  "CAN and LIN Setup " : speedgoatlib_IO611/CAN and LIN Setup   moduleInitValues="[611    1    1   -1   -1]"  id=1  moduleType=IO611  pciSlot=-1  canChn1=CAN (HS)  canChn2=Disabled  canChn3=Disabled  canChn4=Disabled  linChn1=Disabled  linChn2=Disabled  canInitStructArray=[]  canTermStructArray=[]  canChn1InitValues="[2   2   1  31   8   2   1   5   2]"  arbBdrChn1=1.0 MBaud  arbManBdrChn1=[2,1,31,8]  fdBdrChn1=5.0 MBaud  fdManBdrChn1=[2,1,5,2]  canChn2InitValues="[1  200    1   31    8    2    1    5    2]"  arbBdrChn2=10 kBaud  arbManBdrChn2=[200,1,31,8]  fdBdrChn2=5.0 MBaud  fdManBdrChn2=[2,1,5,2]  canChn3InitValues="[1   2   1  31   8   2   1   5   2]"  arbBdrChn3=1.0 MBaud  arbManBdrChn3=[2,1,31,8]  fdBdrChn3=5.0 MBaud  fdManBdrChn3=[2,1,5,2]  canChn4InitValues="[1   2   1  31   8   2   1   5   2]"  arbBdrChn4=1.0 MBaud  arbManBdrChn4=[2,1,31,8]  fdBdrChn4=5.0 MBaud  fdManBdrChn4=[2,1,5,2]  bdrLIN1=19200  linChn1InitValues="[1  19200]"  bdrLIN2=19200  linChn2InitValues="[1  19200]"
      settings: SourceProductName=IO611
  CANPack_ManualSignals : canmsglib/CAN Pack  MsgList=(none)  MsgName=Speed_Cmd  MsgIDType=Standard (11-bit identifier)  MsgIdentifier=0  CANIDInput=off  MsgLength=8  Remote=off  ApplyMinMax=off  BusOutput=on  SignalInfo={ 'Speed_Cmd', '0', '32', 'LE', 'single', 'Standard', '0', '1', '0', '-Inf', 'Inf'; 'Closed_loop', '32', '8', 'LE', 'unsigned', 'Standard', '0', '1', '0', '-Inf', 'Inf'; 'EnablePWM', '40', '8', 'LE', 'unsigned', 'Standard', '0', '1', '0', '-Inf', 'Inf'; 'Filler', '48', '16', 'LE', 'signed', 'Standard', '0', '1', '0', '-Inf', 'Inf' }
      settings: DataFormat=manually specified signals
  CANPack_ManualSignals1 : canmsglib/CAN Pack  MsgList=(none)  MsgName=Speed_Parameters  MsgIDType=Standard (11-bit identifier)  MsgIdentifier=31  CANIDInput=off  MsgLength=8  Remote=off  ApplyMinMax=off  BusOutput=on  SignalInfo={ 'Kp_S', '0', '32', 'LE', 'single', 'Standard', '0', '1', '0', '-Inf', 'Inf'; 'Ki_S', '32', '32', 'LE', 'single', 'Standard', '0', '1', '0', '-Inf', 'Inf' }
      settings: DataFormat=manually specified signals
  CANPack_ManualSignals2 : canmsglib/CAN Pack  MsgList=(none)  MsgName=I_Offsets  MsgIDType=Standard (11-bit identifier)  MsgIdentifier=30  CANIDInput=off  MsgLength=8  Remote=off  ApplyMinMax=off  BusOutput=on  SignalInfo={ 'Ia_offset', '0', '32', 'LE', 'single', 'Standard', '0', '1', '0', '-Inf', 'Inf'; 'Ib_offset', '32', '32', 'LE', 'single', 'Standard', '0', '1', '0', '-Inf', 'Inf' }
      settings: DataFormat=manually specified signals
  CANPack_ManualSignals3 : canmsglib/CAN Pack  MsgList=(none)  MsgName=I_Parameters  MsgIDType=Standard (11-bit identifier)  MsgIdentifier=29  CANIDInput=off  MsgLength=8  Remote=off  ApplyMinMax=off  BusOutput=on  SignalInfo={ 'Kp_I', '0', '32', 'LE', 'single', 'Standard', '0', '1', '0', '-Inf', 'Inf'; 'Ki_I', '32', '32', 'LE', 'single', 'Standard', '0', '1', '0', '-Inf', 'Inf' }
      settings: DataFormat=manually specified signals
  Data Type Conversion : DataTypeConversion  SaturateOnIntegerOverflow=off  RndMeth=Floor
  Gain{,1..3} (4 alike) : Gain
  Mux : Mux
  Pulse Generator : DiscretePulseGenerator  Period=40  PulseWidth=10  SampleTime=Ts_CAN_Tx/10
  Pulse Generator1 : DiscretePulseGenerator  Period=40  PulseWidth=10  PhaseDelay=10  SampleTime=Ts_CAN_Tx/10
  Pulse Generator2 : DiscretePulseGenerator  Period=40  PulseWidth=10  PhaseDelay=20  SampleTime=Ts_CAN_Tx/10
  Pulse Generator3 : DiscretePulseGenerator  Period=40  PulseWidth=10  PhaseDelay=30  SampleTime=Ts_CAN_Tx/10
  Rate Transition{,1..3,5..9} (9 alike) : RateTransition  Integrity=off  Deterministic=off
  Rate Transition4 : RateTransition  Integrity=off  OutPortSampleTime=Ts_CAN_Tx
  Vector Concatenate : Concatenate  NumInputs=4
  Speed_fbk : Outport
  Pos_fdk : Outport  Port=2
  Speed_Cmd : Outport  Port=3
  Spd_pot : Outport  Port=4
  wires:
  "CAN Read "/2 -> CAN Unpack/1
  CAN Unpack/1 -> Speed_fbk/1
  CAN Unpack/2 -> Pos_fdk/1
  "CAN Read "/3 -> CAN Unpack2/1
  CAN Unpack2/2 -> Spd_pot/1
  CAN Unpack2/1 -> Speed_Cmd/1
  Bus Selector/3 -> Rate Transition6/1  "<Kp_S>"
  Bus Selector/4 -> Rate Transition5/1  "<Ki_S>"
  Bus Selector/2 -> Rate Transition1/1  "<Ib_offset>"
  Bus Selector/1 -> Rate Transition/1  "<Ia_offset>"
  Controller_Parameters/1 -> Bus Selector/1
  Bus Selector/6 -> Rate Transition2/1  "<Ki_IxTcpu>"
  Bus Selector/5 -> Rate Transition3/1  "<Kp_I>"
  CANPack_ManualSignals1/1 -> Vector Concatenate/3  "CAN_Ch1_ID102_Tx"
  CANPack_ManualSignals2/1 -> Vector Concatenate/2  "CAN_Ch1_ID102_Tx"
  Pulse Generator/1 -> Gain3/1
  CANPack_ManualSignals/1 -> Vector Concatenate/1  "CAN_Ch1_ID102_Tx"
  Data Type Conversion/1 -> Rate Transition4/1
  Pulse Generator2/1 -> Gain1/1
  Pulse Generator1/1 -> Gain/1
  Mux/1 -> Data Type Conversion/1
  CANPack_ManualSignals3/1 -> Vector Concatenate/4  "CAN_Ch1_ID102_Tx"
  Pulse Generator3/1 -> Gain2/1
  Rate Transition/1 -> CANPack_ManualSignals2/1
  Rate Transition1/1 -> CANPack_ManualSignals2/2
  Rate Transition6/1 -> CANPack_ManualSignals1/1
  Rate Transition5/1 -> CANPack_ManualSignals1/2
  Rate Transition3/1 -> CANPack_ManualSignals3/1
  Rate Transition2/1 -> CANPack_ManualSignals3/2
  Speed_CMD_rpm/1 -> Rate Transition7/1
  Rate Transition7/1 -> CANPack_ManualSignals/1
  Closed_loop/1 -> Rate Transition8/1
  Rate Transition8/1 -> CANPack_ManualSignals/2
  EnablePWM/1 -> Rate Transition9/1
  Rate Transition9/1 -> CANPack_ManualSignals/3
  Gain3/1 -> Mux/1
  Gain/1 -> Mux/2
  Gain1/1 -> Mux/3
  Gain2/1 -> Mux/4
  Vector Concatenate/1 -> "CAN Write "/2
  Rate Transition4/1 -> "CAN Write "/1

== system PMSM3P2LInverterCHILsystem/Three-Phase PMSM System/Controller/Controller_HIL_CAN/Internal PWM configuration1 ==
  Bus Creator1 : BusCreator  Inputs=5
  Not Used Dc : Constant  Value=[0 0 0]  OutDataTypeStr=double
  Not Used Period : Constant  Value=[1 1 1]  OutDataTypeStr=double
  PWM Generation : pwm_cpulib/PWM Generation  f_FPGA=f_FPGA  n_channels=3  sel_scaling=CPU  protection_param=A/B are forced off when A/B are on.  deadband_sec=0  natural_update=At period starts  delay=0  trigger_duration_sec=[1e-6]  trigger_period_start=on  trigger_half_of_the_period=off  trigger_a_on=off  trigger_a_off=off  trigger_b_on=off  trigger_b_off=off  bit_width_pwm_gen=24  invert_a=off  invert_b=on  invert_c=off  showPhaseInput=off
      settings: SourceProductName=PWM CPU Library
  bias4 : Constant  Value=0  OutDataTypeStr=boolean  SampleTime=Ts_UI
  bias5 : Constant  Value=0  OutDataTypeStr=boolean  SampleTime=Ts_UI
  bias6 : Constant  OutDataTypeStr=boolean  SampleTime=Ts_UI
  Simu Config : Outport
  wires:
  PWM Generation/2 -> Bus Creator1/3  "PCIe_PWM_Runtime"
  bias6/1 -> Bus Creator1/5  "PCIe_Protocol"
  PWM Generation/1 -> Bus Creator1/2  "PCIe_PWM_Config"
  Bus Creator1/1 -> Simu Config/1
  bias4/1 -> Bus Creator1/1  "PCIe_RC_or_TTL"
  bias5/1 -> Bus Creator1/4  "PCIe_PWM_Enable"
  Not Used Period/1 -> PWM Generation/1
  Not Used Dc/1 -> PWM Generation/2

== system PMSM3P2LInverterCHILsystem/Three-Phase PMSM System/Controller/Controller_MIL/F28379D ADC ==
  Iab_IO334V : Inport
  Demux : Demux  Outputs=2
  Gain : Gain  Gain=2^12/F28379D_ADC_Vmax
  Ia_ADC : Outport
  Ib_ADC : Outport  Port=2
  wires:
  Iab_IO334V/1 -> Gain/1
  Gain/1 -> Demux/1
  Demux/1 -> Ia_ADC/1
  Demux/2 -> Ib_ADC/1

== system PMSM3P2LInverterCHILsystem/Three-Phase PMSM System/Controller/Controller_MIL/F28379D Firmware ==
  Ia_ADC : Inport
  Ib_ADC : Inport  Port=2
  IaOffset : Inport  Port=3
  IbOffset : Inport  Port=4
  QEP_Position_Count : Inport  Port=5
  QEP_Index_Latch : Inport  Port=6
  SpdCmdRPM : Inport  Port=7
  Kp_S : Inport  Port=8
  Ki_S : Inport  Port=9
  EnClosedLoop : Inport  Port=10
  EnablePWM : Inport  Port=11
  Kp_i : Inport  Port=12
  Ki_ixTcpu : Inport  Port=13
  Controller Algorithm : Subsystem
  Phase_Current_Rescaling : Subsystem
  Speed Conditioning : Subsystem
  ModWave : Outport
  PWM_Enable : Outport  Port=2
  Fbk_CAN : Outport  Port=3
  wires:
  SpdCmdRPM/1 -> Speed Conditioning/1(Spd[rpm])
  Ia_ADC/1 -> Phase_Current_Rescaling/1(Ia_ADC)
  IaOffset/1 -> Phase_Current_Rescaling/3(IaOffset)
  IbOffset/1 -> Phase_Current_Rescaling/4(IbOffset)
  QEP_Position_Count/1 -> Controller Algorithm/2(QEP_Position_Count)
  Controller Algorithm/1(ModWave) -> ModWave/1
  Phase_Current_Rescaling/1(Iab_meas_PU) -> Controller Algorithm/1(Ia_PU)  "Iab_fb_PU"
  Kp_S/1 -> Controller Algorithm/5(Kp_S)
  Controller Algorithm/2(PWM_Enable) -> PWM_Enable/1
  Ki_S/1 -> Controller Algorithm/6(Ki_S)
  QEP_Index_Latch/1 -> Controller Algorithm/3(QEP_Index_Latch)
  Ib_ADC/1 -> Phase_Current_Rescaling/2(Ib_ADC)
  EnClosedLoop/1 -> Controller Algorithm/7(EnClosedLoop)
  EnablePWM/1 -> Controller Algorithm/8(EnablePWM)
  Speed Conditioning/1(Spd[PU]) -> Controller Algorithm/4(SpdCmd)
  Controller Algorithm/3(fbk_CAN) -> Fbk_CAN/1
  Kp_i/1 -> Controller Algorithm/9(Kp_i)
  Ki_ixTcpu/1 -> Controller Algorithm/10(Ki_ixTcpu)

== system PMSM3P2LInverterCHILsystem/Three-Phase PMSM System/Controller/Controller_MIL/IO334 DAC ==
  Iab : Inport
  Add : Sum
  Add Constant : Bias  Bias=[Ia_offset Ib_offset]  SaturateOnIntegerOverflow=off
  Constant : Constant  Value=IO334_iDAC_bias
  Gain : Gain  Gain=IO334_iDAC_gain
  Gain1 : Gain  Gain=2.5/(2^15)
  IO334_DAC_embedded_GAIN : Gain  Gain=2^15/10
  Saturation : Saturate  UpperLimit=IO334_DAC_Vmax  LowerLimit=-IO334_DAC_Vmax
  Iab_IO334DAC : Outport
  wires:
  Iab/1 -> Add Constant/1
  Gain/1 -> Add/1
  Add/1 -> IO334_DAC_embedded_GAIN/1
  Constant/1 -> Add/2
  IO334_DAC_embedded_GAIN/1 -> Gain1/1
  Gain1/1 -> Saturation/1
  Saturation/1 -> Iab_IO334DAC/1
  Add Constant/1 -> Gain/1

== system PMSM3P2LInverterCHILsystem/Three-Phase PMSM System/Three-Phase PMSM Drive/PMSM and average inverter/Encoder Simulation ==
  Theta_m : Inport
  Add1 : Sum  RndMeth=Simplest
  Data Type Conversion7 : DataTypeConversion  OutDataTypeStr=uint16  RndMeth=Simplest  SaturateOnIntegerOverflow=off
  "Get_PU " : Subsystem
  IndexOffset in PU : Constant  Value=0  OutDataTypeStr=single  SampleTime=-1
  Wrap : Subsystem
  pmsm.QEPSlits*4 : Gain  Gain=Maxon_Mile_Nslits*4  OutDataTypeStr=uint16  RndMeth=Simplest
  QEP_Position_Count : Outport
  wires:
  Add1/1 -> Wrap/1(in)
  Theta_m/1 -> "Get_PU "/1(rad)
  pmsm.QEPSlits*4/1 -> Data Type Conversion7/1  "Theta_e"
  Wrap/1(out) -> pmsm.QEPSlits*4/1  "theta_m(ideal)"
  IndexOffset in PU/1 -> Add1/2
  "Get_PU "/1(PU) -> Add1/1
  Data Type Conversion7/1 -> QEP_Position_Count/1

== system PMSM3P2LInverterCHILsystem/Three-Phase PMSM System/Three-Phase PMSM Drive/PMSM and average inverter/Ideal Inverter ==
  V_DC : Inport
  Duty Cycle abc : Inport  Port=2
  Data Type Conversion : DataTypeConversion  OutDataTypeStr=single  SaturateOnIntegerOverflow=off  RndMeth=Floor
  Demux : Demux  Outputs=3
  Mux : Mux  Inputs=3
  Product : Product
  Product1 : Product
  Product2 : Product
  Vabc : Outport
  wires:
  V_DC/1 -> Product2/1, Product1/1, Product/1
  Demux/1 -> Product/2
  Duty Cycle abc/1 -> Data Type Conversion/1
  Mux/1 -> Vabc/1
  Data Type Conversion/1 -> Demux/1
  Demux/2 -> Product1/2
  Demux/3 -> Product2/2
  Product/1 -> Mux/1
  Product1/1 -> Mux/2
  Product2/1 -> Mux/3

== system PMSM3P2LInverterCHILsystem/Three-Phase PMSM System/Three-Phase PMSM Drive/PMSM and average inverter/PMSM ==
  Config : Inport
  PhaseVolt abc : Inport  Port=2
  LdTrq / Spd : Inport  Port=3
  Constant : Constant  Value=0  OutDataTypeStr=boolean
  PMSM HDL : mcbhdlplantlib/PMSM HDL  VariantControl=pmsmVariant==pmsmEnum.TorqueInput  Ts=Ts_CPU  dataTypePop=Floating-point  Imax=21  CurrWordLen=32  Nmax=4000*4*(2*pi/60)  NWordLen=32  Tmax=0.27*2  TWordLen=32  Tbl={'Max Current (A)','fixdt(1,32,26)','-32','32','3.4694e-18';'Max Electrical Speed (Rad/s)','fixdt(1,32,20)','-2048','2048','1.4552e-11';'Max Torque (NM)','fixdt(1,32,31)','-1','1','4.6566e-10'}
      settings: LibrarySourceBlock=mcbhdllib/Electrical Systems/Motors/PMSM HDL
  Info : Outport
  PhaseCurr : Outport  Port=2
  Torque : Outport  Port=3
  RotorMechSpd : Outport  Port=4
  RotorElecAngle : Outport  Port=5
  wires:
  PMSM HDL/5 -> RotorElecAngle/1
  Config/1 -> PMSM HDL/1
  PMSM HDL/4 -> RotorMechSpd/1
  PMSM HDL/3 -> Torque/1
  PMSM HDL/2 -> PhaseCurr/1
  LdTrq / Spd/1 -> PMSM HDL/3
  PhaseVolt abc/1 -> PMSM HDL/2
  PMSM HDL/1 -> Info/1
  Constant/1 -> PMSM HDL/4

== system PMSM3P2LInverterCHILsystem/Three-Phase PMSM System/Three-Phase PMSM Drive/PMSM and average inverter/Runtime to DC ==
  PWM_Runtime : Inport
  Demux : Demux  Outputs=15
  Mux : Mux  Inputs=3
  To Dc A1 : Subsystem
  To Dc A2 : Subsystem
  To Dc A3 : Subsystem
  Duty Cycle abc : Outport
  wires:
  PWM_Runtime/1 -> Demux/1  "PCIe_PWM_Runtime"
  Demux/2 -> To Dc A1/1(A_on)
  Demux/3 -> To Dc A1/2(A_off)
  Demux/7 -> To Dc A2/1(A_on)
  Demux/8 -> To Dc A2/2(A_off)
  Demux/12 -> To Dc A3/1(A_on)
  Demux/13 -> To Dc A3/2(A_off)
  To Dc A1/1(Dc) -> Mux/1
  To Dc A2/1(Dc) -> Mux/2
  To Dc A3/1(Dc) -> Mux/3
  Mux/1 -> Duty Cycle abc/1

== system PMSM3P2LInverterCHILsystem/Three-Phase PMSM System/Three-Phase PMSM Drive/PMSM and inverter with switching dynamics/DAC Config ==
  Gain : Gain
  I DAC bias : Constant  Value=IO334_iDAC_bias  OutDataTypeStr=single  SampleTime=Ts_UI
  I DAC gain : Constant  Value=IO334_iDAC_gain  OutDataTypeStr=single  SampleTime=Ts_UI
  Plant_Prequency : Constant  Value=1/ts_FPGA_mdl  SampleTime=Ts_UI
  Sig_frequ : Constant  Value=100000  VectorParams1D=off  SampleTime=Ts_UI
  Subsystem : Subsystem
  I_DAC_gain : Outport
  I_DAC_Current : Outport  Port=2
  DAC_reset : Outport  Port=3
  wires:
  Subsystem/1(DAC_reset) -> DAC_reset/1
  Plant_Prequency/1 -> Subsystem/1(Plant_frequency)
  Sig_frequ/1 -> Subsystem/2(SignalFrequency)
  I DAC bias/1 -> I_DAC_Current/1
  I DAC gain/1 -> Gain/1
  Gain/1 -> I_DAC_gain/1

== system PMSM3P2LInverterCHILsystem/Three-Phase PMSM System/Three-Phase PMSM Drive/PMSM and inverter with switching dynamics/Encoder Simulation ==
  Theta_m : Inport
  Add1 : Sum  RndMeth=Simplest
  Data Type Conversion7 : DataTypeConversion  OutDataTypeStr=uint16  RndMeth=Simplest  SaturateOnIntegerOverflow=off
  "Get_PU " : Subsystem
  IndexOffset in PU : Constant  Value=0  OutDataTypeStr=single  SampleTime=-1
  Wrap : Subsystem
  pmsm.QEPSlits*4 : Gain  Gain=Maxon_Mile_Nslits*4  OutDataTypeStr=uint16  RndMeth=Simplest
  QEP_Position_Count : Outport
  wires:
  Add1/1 -> Wrap/1(in)
  Theta_m/1 -> "Get_PU "/1(rad)
  pmsm.QEPSlits*4/1 -> Data Type Conversion7/1  "Theta_e"
  Wrap/1(out) -> pmsm.QEPSlits*4/1  "theta_m(ideal)"
  IndexOffset in PU/1 -> Add1/2
  "Get_PU "/1(PU) -> Add1/1
  Data Type Conversion7/1 -> QEP_Position_Count/1

== system PMSM3P2LInverterCHILsystem/Three-Phase PMSM System/Three-Phase PMSM Drive/PMSM and inverter with switching dynamics/PMSM Configuration ==
  Inertia : Constant  Value=J  OutDataTypeStr=single  SampleTime=Ts
  Mux : Mux  Inputs=9
  Number of pole pairs : Constant  Value=Pp  OutDataTypeStr=single  SampleTime=Ts
  Permanent magnet flux linkage : Constant  Value=lambda_pm  OutDataTypeStr=single  SampleTime=Ts
  Static friction : Constant  Value=f  OutDataTypeStr=single  SampleTime=Ts
  Stator d-axis inductance : Constant  Value=Ld  OutDataTypeStr=single  SampleTime=Ts
  Stator q-axis inductance : Constant  Value=Lq  OutDataTypeStr=single  SampleTime=Ts
  Stator resistance per phase : Constant  Value=Rs  OutDataTypeStr=single  SampleTime=Ts
  TrqSpdCtrl : Constant  Value=Trq_N_mode  OutDataTypeStr=single  SampleTime=Ts
  Viscous damping : Constant  Value=B  OutDataTypeStr=single  SampleTime=Ts
  PCIe_Motor_Config : Outport
  wires:
  Permanent magnet flux linkage/1 -> Mux/5
  Stator resistance per phase/1 -> Mux/2
  TrqSpdCtrl/1 -> Mux/9
  Static friction/1 -> Mux/8
  Viscous damping/1 -> Mux/7
  Mux/1 -> PCIe_Motor_Config/1
  Inertia/1 -> Mux/6
  Stator q-axis inductance/1 -> Mux/4
  Stator d-axis inductance/1 -> Mux/3
  Number of pole pairs/1 -> Mux/1
